simulink model "UniTire_0427_2021b_PID"  (R2021b)
settings: Solver=FixedStepAuto  StartTime=0.0  StopTime=15  FixedStep=0.001  RelTol=1e-3
model workspace (MAT data in the model file):
  v_obj = Simulink.Parameter
  v_obj.DataType = 'auto'
  v_obj.Complexity = 'real'
  v_obj.Dimensions = [0 0]
libraries: Solver_SF x1, slpidlib x1
settings Model: Creator=11580  LastModifiedBy=user
settings SolverCC: ZeroCrossAlgorithm=Adaptive
settings DebuggingCC: IgnoredZcDiagnostic=none  UnconnectedInputMsg=none  UnconnectedOutputMsg=none  UnconnectedLineMsg=none
settings ModelReferenceCC: EnableRefExpFcnMdlSchedulingChecks=off
settings RTWCC: DLArmComputeVersion=20.02.1

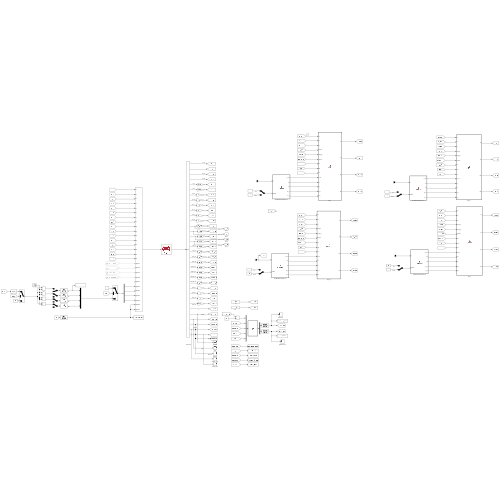
[thumbnail: Simulink's stored preview of the top-level diagram]
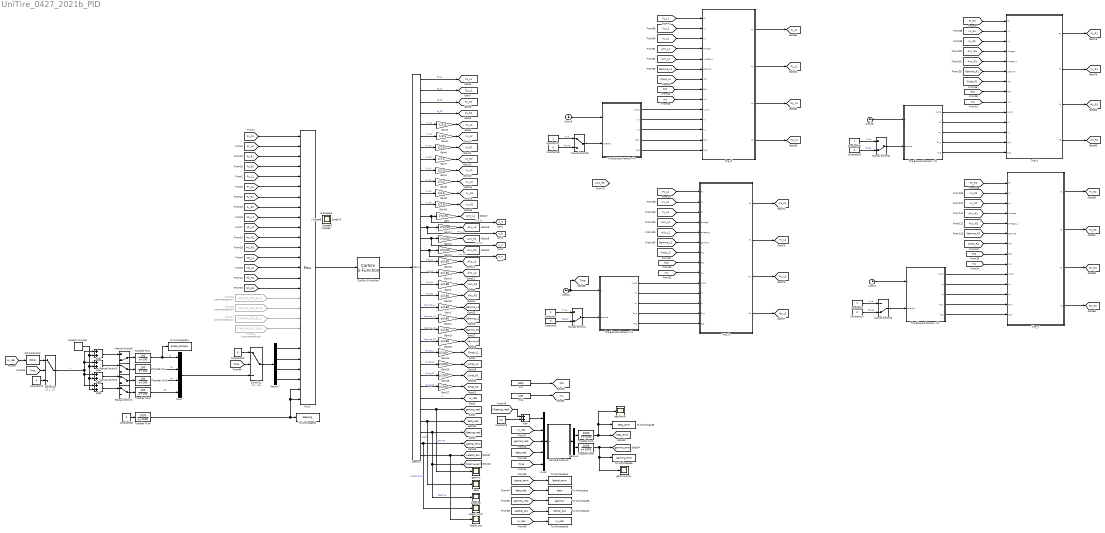
== system UniTire_0427_2021b_PID ==
  Add{,1..4} (5 alike) : Sum
  CarSim S-Function : Solver_SF/CarSim S-Function  Priority=1  SIMFILE=simfile.sim  Run_RTs=off  vs_state_ind=Run  StopMode_ind=Vehicle Model
  Clock{1..2,8..9} (4 alike) : Clock
  Constant{1..2,15,17} (4 alike) : Constant
  Constant{3,10,16,18,20..21,25} (7 alike) : Constant  Value=0
  Constant9 : Constant  Value=0.2
  Demux : Demux  Outputs=34
      settings: DisplayOption=none
  Demux1 : Demux  Outputs=2
  Demux7 : Demux
  From12 : From  Commented=on  GotoTag=IMP_MY_OUT_D2_R
  From17 : From  Commented=on  GotoTag=IMP_MY_OUT_D2_L
  From20 : From  Commented=on  GotoTag=IMP_MY_OUT_D1_R
  From21 : From  Commented=on  GotoTag=IMP_MY_OUT_D1_L
  Fzn : Constant  Value=4820
  Gain{,11..13} (4 alike) : Gain  Gain=2*pi/60
  Gain{1..2,14..19} (8 alike) : Gain  Gain=pi/180
  Gain{3..10} (8 alike) : Gain  Gain=1/3.6
  Gain{24..27} (4 alike) : Gain  Gain=1/1000
  MATLAB Function : MATLAB Function  TreatAsAtomicUnit=on
  Manual Switch{1,5..6,8} (4 alike) : ManualSwitch  CurrentSetting=0
  Manual Switch{2..4,9} (4 alike) : ManualSwitch
  Mux2 : Mux  Inputs=27
      settings: DisplayOption=signals
  Mux5 : Mux  Inputs=5
  Mux7 : Mux
  PID Controller : slpidlib/PID Controller  Controller=PID  Form=Parallel  TimeDomain=Continuous-time  UseExternalTs=off  SampleTime=-1  IntegratorMethod=Forward Euler  FilterMethod=Forward Euler  ControllerParametersSource=internal  P=4  I=0  D=1  UseFilter=on  N=100  TunerSelectOption=Transfer Function Based (PID Tuner App)  InitialConditionSource=internal  InitialConditionForIntegrator=0  InitialConditionForFilter=0  DifferentiatorICPrevScaledInput=0  ExternalReset=none  TrackingMode=off  Kt=1  LimitOutput=off  SatLimitsSource=internal  UpperSaturationLimit=inf  LowerSaturationLimit=-inf  LinearizeAsGain=on  AntiWindupMode=none  Kb=1  POutMin=[]  POutMax=[]  IOutMin=[]  IOutMax=[]  DOutMin=[]  DOutMax=[]  NOutMin=[]  NOutMax=[]  SumOutMin=[]  SumOutMax=[]  SaturationOutMin=[]  SaturationOutMax=[]  PParamMin=[]  PParamMax=[]  IParamMin=[]  IParamMax=[]  DParamMin=[]  DParamMax=[]  NParamMin=[]  NParamMax=[]  KbParamMin=[]  KbParamMax=[]  KtParamMin=[]  KtParamMax=[]  KbOutMin=[]  KbOutMax=[]  KtOutMin=[]  KtOutMax=[]  IntegratorOutMin=[]  IntegratorOutMax=[]  FilterOutMin=[]  FilterOutMax=[]  SumI1OutMin=[]  SumI1OutMax=[]  SumI2OutMin=[]  SumI2OutMax=[]  SumI3OutMin=[]  SumI3OutMax=[]  SumI4OutMin=[]  SumI4OutMax=[]  SumDOutMin=[]  SumDOutMax=[]  DifferentiatorOutMin=[]  DifferentiatorOutMax=[]  FilterDiffOutCoefMin=[]  FilterDiffOutCoefMax=[]  ReciprocalOutMin=[]  ReciprocalOutMax=[]  SumDenOutMin=[]  SumDenOutMax=[]  SumNumOutMin=[]  SumNumOutMax=[]  DivideOutMin=[]  DivideOutMax=[]  UdiffTsProdOutMin=[]  UdiffTsProdOutMax=[]  NTsProdOutMin=[]  NTsProdOutMax=[]  UintegralTsProdOutMin=[]  UintegralTsProdOutMax=[]  UngainTsProdOutMin=[]  UngainTsProdOutMax=[]  IntegratorContinuousStateAttributes=''  IntegratorStateMustResolveToSignalObject=off  IntegratorRTWStateStorageClass=Auto  FilterContinuousStateAttributes=''  FilterStateMustResolveToSignalObject=off  FilterRTWStateStorageClass=Auto  ParallelPVariant=InternalParameters  IdealPVariant=Disabled  IVariant=InternalParameters  DVariant=InternalParameters  IntegratorVariant=Continuous  SatVariant=Disabled  AWVariant=Passthrough  PCopyVariant=Disabled  TRVariant=Disabled  FdbkBlocksVariant=Forward  IdealPFdbkVariant=Disabled  SatFdbkVariant=Disabled  DerivativeFilterVariant=ContFilter  NVariant=InternalParameters  NCopyVariant=Disabled  FilterICVariant=InternalICsFilter  IntegratorICVariant=InternalICs  ExternalResetVariant=Disabled  TRSumVariant=Passthrough  SumFdbkVariant=Disabled  SumVariant=Sum_PID  TsampFilterVariant=InternalTs  TsampNgainVariant=Passthrough  TsampIntegralVariant=Passthrough  ExternalSaturationOutDataTypeStr=Inherit: Same as second input
  Random Number : RandomNumber  Variance=150  SampleTime=0.01
  Switch10 : Switch  Criteria=u2 > Threshold  Threshold=1.5
  Switch11 : Switch  Criteria=u2 > Threshold  Threshold=15
  Tire Blowout Params. rl1 : MATLAB Function  TreatAsAtomicUnit=on
  Tire Blowout Params. rl2 : MATLAB Function  TreatAsAtomicUnit=on
  Tire Blowout Params. rl3 : MATLAB Function  TreatAsAtomicUnit=on
  Tire Blowout Params. rl4 : MATLAB Function  TreatAsAtomicUnit=on
  Tire_fl : MATLAB Function  TreatAsAtomicUnit=on
  Tire_fr : MATLAB Function  TreatAsAtomicUnit=on
  Tire_rl1 : MATLAB Function  TreatAsAtomicUnit=on
  Tire_rr : MATLAB Function  TreatAsAtomicUnit=on
  To Workspace : ToWorkspace  VariableName=beta  SaveFormat=Timeseries  SampleTime=-1
  To Workspace1 : ToWorkspace  VariableName=lateral_error  SaveFormat=Timeseries  SampleTime=-1
  To Workspace11 : ToWorkspace  VariableName=Brake_torque1  SaveFormat=Timeseries  SampleTime=-1
  To Workspace2 : ToWorkspace  VariableName=Steering  SaveFormat=Timeseries  SampleTime=-1
  To Workspace3 : ToWorkspace  VariableName=gamma  SaveFormat=Timeseries  SampleTime=-1
  To Workspace4 : ToWorkspace  VariableName=lateral_acc  SaveFormat=Timeseries  SampleTime=-1
  To Workspace5 : ToWorkspace  VariableName=vx_real  SaveFormat=Timeseries  SampleTime=-1
  To Workspace8 : ToWorkspace  VariableName=beta_error  SaveFormat=Timeseries  SampleTime=-1
  To Workspace9 : ToWorkspace  VariableName=gamma_error  SaveFormat=Timeseries  SampleTime=-1
  Transfer Fcn{,1..3} (4 alike) : TransferFcn  Numerator=[100]  Denominator=[1 100]
  Transfer Fcn4 : TransferFcn  Numerator=[1000]  Denominator=[1 1000]
  Transfer Fcn5 : TransferFcn  Numerator=[1000]  Denominator=[1 1000]
  Transfer Fcn6 : TransferFcn  Numerator=[1000]  Denominator=[1 1000]
  beta : Scope
  beta error : Scope
  gamma : Scope
  gamma error : Scope
  lateral_acc : Scope
  lateral_error : Scope
  mu1 : Constant  Value=0.85
  steering : Scope
  Scope{,1..9,11..12,14,16,19..23,25..26} (21 alike) : Scope
  tag scope: AVy_L1=global, AVy_L2=global, AVy_R1=global, AVy_R2=global, AVz_L1=global, AVz_L2=global, AVz_R1=global, AVz_R2=global, Cmpt_L1=global, Cmpt_L2=global, Cmpt_R1=global, Cmpt_R2=global, Fx_L1=global, Fx_L2=global, Fx_R1=global, Fx_R2=global, Fy_L1=global, Fy_L2=global, Fy_R1=global, Fy_R2=global, Fz0=global, Fz_L1=global, Fz_L2=global, Fz_R1=global, Fz_R2=global, Gamma_L1=global, Gamma_L2=global, Gamma_R1=global, Gamma_R2=global, Lateral_acc=global, Lateral_error=global, My_L1=global, My_L2=global, My_R1=global, My_R2=global, Mz_L1=global, Mz_L2=global, Mz_R1=global, Mz_R2=global, Steering_real=global, Time=global, Vx_L1=global, Vx_L2=global, Vx_R1=global, Vx_R2=global, Vy_L1=global, Vy_L2=global, Vy_R1=global, Vy_R2=global, beta_error=global, beta_real=global, gamma_error=global, gamma_real=global, mu=global, n_fl=global, n_fr=global, n_rl=global, n_rr=global, vx_real=global
  wires:
  Demux/5 -> Gain3/1  "Vx_L1"
  Demux/13 -> [n_fl], Gain/1  "AVy_L1"
  Demux/17 -> Gain15/1  "AVz_L1"
  Demux/21 -> Gain1/1  "Gamma_L1"
  Demux/25 -> Gain24/1  "Cmpt_L1"
  Gain3/1 -> [Vx_L1]
  Demux/1 -> [Fz_L1]  "Fz_L1"
  Demux/2 -> [Fz_L2]  "Fz_L2"
  Demux/3 -> [Fz_R1]  "Fz_R1"
  Demux/4 -> [Fz_R2]  "Fz_R2"
  Demux/6 -> Gain5/1  "Vx_L2"
  Gain5/1 -> [Vx_L2]
  Demux/7 -> Gain6/1  "Vx_R1"
  Gain6/1 -> [Vx_R1]
  Demux/8 -> Gain7/1  "Vx_R2"
  Gain7/1 -> [Vx_R2]
  Gain4/1 -> [Vy_L1]
  Demux/9 -> Gain4/1  "Vy_L1"
  Gain8/1 -> [Vy_L2]
  Demux/10 -> Gain8/1  "Vy_L2"
  Gain9/1 -> [Vy_R1]
  Demux/11 -> Gain9/1  "Vy_R1"
  Gain10/1 -> [Vy_R2]
  Demux/12 -> Gain10/1  "Vy_R2"
  Gain/1 -> [AVy_L1]
  Gain11/1 -> [AVy_L2]
  Demux/14 -> [n_fr], Gain11/1  "AVy_L2"
  Gain12/1 -> [AVy_R1]
  Demux/15 -> [n_rl], Gain12/1  "AVy_R1"
  Gain13/1 -> [AVy_R2]
  Demux/16 -> [n_rr], Gain13/1  "AVy_R2"
  Demux/18 -> Gain14/1  "AVz_L2"
  Demux/19 -> Gain2/1  "AVz_R1"
  Demux/20 -> Gain16/1  "AVz_R2"
  Gain16/1 -> [AVz_R2]
  Gain1/1 -> [Gamma_L1]
  Gain17/1 -> [Gamma_L2]
  Demux/22 -> Gain17/1  "Gamma_L2"
  Gain18/1 -> [Gamma_R1]
  Demux/23 -> Gain18/1  "Gamma_R1"
  Gain19/1 -> [Gamma_R2]
  Demux/24 -> Gain19/1  "Gamma_R2"
  Gain2/1 -> [AVz_R1]
  Gain14/1 -> [AVz_L2]
  Gain15/1 -> [AVz_L1]
  Demux/26 -> Gain25/1  "Cmpt_21"
  Demux/27 -> Gain26/1  "Cmpt_R1"
  Demux/28 -> Gain27/1  "Cmpt_R2"
  Demux/29 -> [vx_real]  "Vx"
  [mu] -> Tire_rl1/9(mu)
  [Fz0] -> Tire_fr/8(Fz0)
  [Gamma_R1] -> Tire_fr/6(gamma)
  Tire_fr/4(Mz) -> [Mz_R1]
  [Fz_L1] -> Tire_fl/1(Fz)
  mu1/1 -> [mu]
  Tire_rl1/3(My) -> [My_L2]
  [AVy_L2] -> Tire_rl1/4(Omega)
  [AVz_R2] -> Tire_rr/5(omega_z)
  [Fz0] -> Tire_rr/8(Fz0)
  Fzn/1 -> [Fz0]
  [Gamma_R2] -> Tire_rr/6(gamma)
  Tire_fr/1(Fx) -> [Fx_R1]
  [Vx_R1] -> Tire_fr/2(Vx)
  [AVy_R2] -> Tire_rr/4(Omega)
  Tire_rr/1(Fx) -> [Fx_R2]
  Tire_rl1/4(Mz) -> [Mz_L2]
  [mu] -> Tire_rr/9(mu)
  [Cmpt_R2] -> Tire_rr/7(rho)
  [Vx_L2] -> Tire_rl1/2(Vx)
  Tire_fl/4(Mz) -> [Mz_L1]
  [Vx_R2] -> Tire_rr/2(Vx)
  [AVz_L2] -> Tire_rl1/5(omega_z)
  [mu] -> Tire_fl/9(mu)
  [AVz_L1] -> Tire_fl/5(omega_z)
  [Gamma_L1] -> Tire_fl/6(gamma)
  [AVy_R1] -> Tire_fr/4(Omega)
  Tire_rr/3(My) -> [My_R2]
  [Fz_R1] -> Tire_fr/1(Fz)
  [Gamma_L2] -> Tire_rl1/6(gamma)
  Tire_rr/4(Mz) -> [Mz_R2]
  [Cmpt_L2] -> Tire_rl1/7(rho)
  Tire_fl/3(My) -> [My_L1]
  [Fz0] -> Tire_rl1/8(Fz0)
  Tire_rl1/1(Fx) -> [Fx_L2]
  Tire_fl/1(Fx) -> [Fx_L1]
  [mu] -> Tire_fr/9(mu)
  [Fz_L2] -> Tire_rl1/1(Fz)
  [Vy_L2] -> Tire_rl1/3(Vy)
  [Fz_R2] -> Tire_rr/1(Fz)
  Tire_fr/3(My) -> [My_R1]
  [Vy_R1] -> Tire_fr/3(Vy)
  [Vy_R2] -> Tire_rr/3(Vy)
  [AVz_R1] -> Tire_fr/5(omega_z)
  [Fz0] -> Tire_fl/8(Fz0)
  [Cmpt_L1] -> Tire_fl/7(rho)
  [Cmpt_R1] -> Tire_fr/7(rho)
  [AVy_L1] -> Tire_fl/4(Omega)
  [Vy_L1] -> Tire_fl/3(Vy)
  From21/1 -> Mux2/17
  [My_R1] -> Mux2/11
  From12/1 -> Mux2/20
  [Mz_R2] -> Mux2/16
  [My_L2] -> Mux2/10
  [Fx_L2] -> Mux2/2
  [Fx_R2] -> Mux2/4
  [Fy_L1] -> Mux2/5
  [Fy_R1] -> Mux2/7
  [Fy_R2] -> Mux2/8
  [My_L1] -> Mux2/9
  [My_R2] -> Mux2/12
  [Mz_L2] -> Mux2/14
  [Fx_R1] -> Mux2/3
  From20/1 -> Mux2/18
  [Mz_R1] -> Mux2/15
  [Mz_L1] -> Mux2/13
  From17/1 -> Mux2/19
  [Fy_L2] -> Mux2/6
  [Fx_L1] -> Mux2/1
  [Vx_L1] -> Tire_fl/2(Vx)
  Gain24/1 -> [Cmpt_L1]
  Gain25/1 -> [Cmpt_L2]
  Gain26/1 -> [Cmpt_R1]
  Gain27/1 -> [Cmpt_R2]
  Tire Blowout Params. rl2/5(R_e) -> Tire_rr/14(R_e)
  Tire Blowout Params. rl2/4(Rr_c) -> Tire_rr/13(Rr_c)
  Tire Blowout Params. rl2/3(Ky) -> Tire_rr/12(Ky)
  Tire Blowout Params. rl2/2(Kx) -> Tire_rr/11(Kx)
  Tire Blowout Params. rl2/1(K_rho) -> Tire_rr/10(K_rho)
  Constant1/1 -> Manual Switch5/1  "True"
  Clock1/1 -> Tire Blowout Params. rl2/1(t)
  Constant10/1 -> Manual Switch5/2  "fause"
  Manual Switch5/1 -> Tire Blowout Params. rl2/2(enable)
  Manual Switch8/1 -> Tire Blowout Params. rl3/2(enable)
  Constant16/1 -> Manual Switch8/2  "fause"
  Clock8/1 -> Tire Blowout Params. rl3/1(t)
  Constant15/1 -> Manual Switch8/1  "True"
  Tire Blowout Params. rl3/1(K_rho) -> Tire_fr/10(K_rho)
  Tire Blowout Params. rl3/2(Kx) -> Tire_fr/11(Kx)
  Tire Blowout Params. rl3/3(Ky) -> Tire_fr/12(Ky)
  Tire Blowout Params. rl3/4(Rr_c) -> Tire_fr/13(Rr_c)
  Tire Blowout Params. rl3/5(R_e) -> Tire_fr/14(R_e)
  Tire Blowout Params. rl4/5(R_e) -> Tire_fl/14(R_e)
  Tire Blowout Params. rl4/4(Rr_c) -> Tire_fl/13(Rr_c)
  Tire Blowout Params. rl4/3(Ky) -> Tire_fl/12(Ky)
  Tire Blowout Params. rl4/2(Kx) -> Tire_fl/11(Kx)
  Tire Blowout Params. rl4/1(K_rho) -> Tire_fl/10(K_rho)
  Constant17/1 -> Manual Switch9/1  "True"
  Clock9/1 -> Tire Blowout Params. rl4/1(t)
  Constant18/1 -> Manual Switch9/2  "fause"
  Manual Switch9/1 -> Tire Blowout Params. rl4/2(enable)
  Manual Switch1/1 -> Tire Blowout Params. rl1/2(enable)
  Constant3/1 -> Manual Switch1/2  "fause"
  Clock2/1 -> [Time], Tire Blowout Params. rl1/1(t)
  Constant2/1 -> Manual Switch1/1  "True"
  Tire Blowout Params. rl1/1(K_rho) -> Tire_rl1/10(K_rho)
  Tire Blowout Params. rl1/2(Kx) -> Tire_rl1/11(Kx)
  Tire Blowout Params. rl1/3(Ky) -> Tire_rl1/12(Ky)
  Tire Blowout Params. rl1/4(Rr_c) -> Tire_rl1/13(Rr_c)
  Tire Blowout Params. rl1/5(R_e) -> Tire_rl1/14(R_e)
  Demux/30 -> [gamma_real], gamma/1  "gamma"
  Mux5/1 -> MATLAB Function/1(u)
  Demux/32 -> [Steering_real], steering/1, [Steering_real]  "steering"
  Demux/31 -> [beta_real], beta/1  "beta"
  [vx_real] -> Mux5/2
  [gamma_real] -> Mux5/3
  [beta_real] -> Mux5/4
  MATLAB Function/1(y) -> Demux1/1
  Demux1/1 -> Transfer Fcn5/1
  Demux1/2 -> Transfer Fcn6/1
  Demux/33 -> [Lateral_error], lateral_error/1  "lateral error"
  [Time] -> Switch10/2
  Demux/34 -> lateral_acc/1, [Lateral_acc]
  [beta_real] -> To Workspace/1
  [gamma_real] -> To Workspace3/1
  [Lateral_error] -> To Workspace1/1
  [Lateral_acc] -> To Workspace4/1
  [vx_real] -> To Workspace5/1
  Transfer Fcn/1 -> Mux7/2  "LR"
  Transfer Fcn1/1 -> Mux7/1, To Workspace11/1  "LF"
  Transfer Fcn2/1 -> Mux7/3  "RF"
  Transfer Fcn3/1 -> Mux7/4  "RR"
  Manual Switch2/1 -> Transfer Fcn3/1
  Manual Switch3/1 -> Transfer Fcn/1
  Manual Switch4/1 -> Transfer Fcn2/1
  Manual Switch6/1 -> Transfer Fcn1/1
  Mux7/1 -> Switch11/3
  [Time] -> Mux5/5
  Add/1 -> Mux5/1
  [Steering_real] -> Add/1
  Constant9/1 -> Add/2
  Transfer Fcn4/1 -> To Workspace2/1, Mux2/27, Mux2/26
  Transfer Fcn5/1 -> beta error/1, To Workspace8/1, [beta_error]
  Transfer Fcn6/1 -> To Workspace9/1, gamma error/1, [gamma_error]
  Tire_rl1/2(Fy) -> [Fy_L2]
  Tire_rr/2(Fy) -> [Fy_R2]
  Tire_fr/2(Fy) -> [Fy_R1]
  Tire_fl/2(Fy) -> [Fy_L1]
  [vx_real] -> PID Controller/1
  Mux2/1 -> CarSim S-Function/1
  CarSim S-Function/1 -> Demux/1
  Switch10/1 -> Add4/1, Add3/1, Add1/1, Add2/1  "1"
  PID Controller/1 -> Switch10/1
  Constant21/1 -> Switch10/3
  Add1/1 -> Manual Switch6/1
  Random Number/1 -> Add4/2, Add3/2, Add2/2, Add1/2
  Add2/1 -> Manual Switch3/1
  Add3/1 -> Manual Switch4/1
  Add4/1 -> Manual Switch2/1
  Demux7/1 -> Mux2/22
  Demux7/2 -> Mux2/23
  Demux7/3 -> Mux2/24
  Demux7/4 -> Mux2/25
  [Time] -> Switch11/2
  Constant20/1 -> Switch11/1
  Switch11/1 -> Demux7/1
  Constant25/1 -> Transfer Fcn4/1

== matlab function UniTire_0427_2021b_PID/Tire Blowout Params. rl4 ==
  data: K_rho output; Kx output; Ky output; Rr_c output; R_e output; t input; enable input
function [K_rho, Kx, Ky, Rr_c, R_e] = TireBlowout(t, enable)
% 初始参数
K_rho0 = 268000;     % Radial stiffness (N/m)
Kx0 = 1586.04;       % Longitudinal stiffness (N/unit slip)
Ky0 = 63430.51;      % Lateral stiffness (N/rad)
Rr_c0 = 0.0038;      % Rolling resistance coefficient
R_e0 = 0.325;        % Effective rolling radius

% 如果 enable<=0.5，始终输出初始参数
K_rho    = K_rho0;
Kx       = Kx0;
Ky       = Ky0;
Rr_c     = Rr_c0;
R_e      = R_e0;

   if enable > 0.5
       % 爆胎开始时间与过渡时长
       t_start    = 1;   % 3 s 开始
       t_duration = 0.1;   % 持续 100 ms
   
       % 计算过渡比例 t_ratio
       if     t <  t_start
              t_ratio = 0;
          elseif  t <= t_start + t_duration
              t_ratio = (t - t_start) / t_duration;
          else
              t_ratio = 1;    % 过渡完成后一直保持
       end
   
       % Define blowout parameter factors
       K_rho_factor    = 1/15;   % Reduce radial stiffness to 1/15
       Kx_factor       = 0.28;   % Reduce longitudinal stiffness to 28%
       Ky_factor       = 0.25;   % Reduce lateral stiffness to 25%
       Rr_c_factor     = 30;     % Increase rolling resistance by 30x
       R_e_factor      = 0.7;    % Reduce effective radius to 70%
   
       % 按 t_ratio 做线性插值
       K_rho    = K_rho0 * (1 - t_ratio) + (K_rho0 * K_rho_factor) * t_ratio;
       Kx       = Kx0 * (1 - t_ratio) + (Kx0 * Kx_factor) * t_ratio;
       Ky       = Ky0 * (1 - t_ratio) + (Ky0 * Ky_factor) * t_ratio;
       Rr_c     = Rr_c0 * (1 - t_ratio) + (Rr_c0 * Rr_c_factor) * t_ratio;
       R_e      = R_e0 * (1 - t_ratio) + (R_e0 * R_e_factor) * t_ratio;
   end

end

== matlab function UniTire_0427_2021b_PID/Tire_fl ==
  data: Fz input; Vx input; Fx output; Vy input; Omega input; omega_z input; gamma input; rho input; Fz0 input; mu input; K_rho input; Kx input; Ky input; Rr_c input; R_e input; Fy output; My output; Mz output
function [Fx, Fy, My, Mz] = UniTire_fl(Fz, Vx, Vy, Omega, omega_z, gamma, rho, Fz0, mu, K_rho, Kx, Ky, Rr_c, R_e)
%% 解析轮胎参数       
a1      = 0.02;  % 接地印迹半长经验系数1
a2      = 0.001; % 接地印迹半长经验系数2
lambda  = 1.00;  % 各向异性修正系数 
eps_val = 1e-12;
    
%% 计算
% 1.垂向力Fz
% Fz = K_rho * rho;
Fzn = Fz / Fz0; % 归一化垂向力

% 接地印迹半长
a = a1 * sqrt(max(Fz, 0)) + a2 * max(Fz, 0);

% 2.滑移率和刚度计算
    if abs(Omega) < eps_val
        Omega_safe = eps_val * sign(Omega + eps_val);  % Defaults to positive when Omega is exactly 0
    else
        Omega_safe = Omega;
    end

Sx = (Omega_safe * R_e - Vx) / (Omega_safe * R_e);  % 纵向滑移率
Sy = -Vy / (Omega_safe * R_e);                      % 侧向滑移率

%Sy_cam = -(Ky_gamma * sin(gamma)) / max(Ky, eps_val);
%Sy = Sy0 + Sy_cam; 

% 纵向及侧向的摩擦系数
%Ux = (Fzn^2 * (mu*(-0.048735)/0.345728)) + (Fzn*(mu*0.048084/0.345728)) + mu;
Ux = mu;
Uy = mu;

% 无量纲的相对滑移率
phi_X = (Sx * Kx) / max(Fz * Ux, eps_val);
phi_Y = (Sy * Ky) / max(Fz * Uy, eps_val);
phi = sqrt(phi_X.^2 + phi_Y.^2);

% 5.计算总切力因子 F
c1 = 15.804511^2; c2 = 13.644270^2; c3 = 132.496949; c4 = 8.120481;
E1 = 1 ./ ( exp(-Fzn / c1) * c2 + 2 );
Em = 1 ./ ( 2 + c3^2 * exp(-Fzn/c4^2) );

F = 1 - exp( -phi - ( phi^3 * (E1^2 + 1/12) + E1 * phi^2 ) );

% 计算纵向力部分
F_x = F * (phi_X / phi);
Fx = Fz * F_x * Ux;

% 计算侧向力部分
F_y = F * (phi_Y / phi);
Fy = Fz * F_y * Uy;

% 6.回正力矩计算
% 计算Kxc和Kyc
Kxc = 100548.546 * Fzn + 52024.374 * (Fzn^2); % 胎体纵向刚度 (N/m)
Kyc = 100548.546 * Fzn + 52024.374 * (Fzn^2); % 胎体侧向刚度 (N/m)

    % 限制最小刚度值
    Kxc = max(Kxc, 1000); % 最小刚度1kN/m
    Kyc = max(Kyc, 1000);
    
% 计算Dx参数
Dx0 = (-0.013812)*(Fzn^2) + 0.007221*Fzn - 0.025351;
De  = (-0.008474)*(Fzn^2) + 0.022706*Fzn - 0.005839;
D1 = 1.168453 * exp(-Fzn / 1.008694);  % 曲率因子1
D2 = 0.018910 * exp(-Fzn / 0.663584);  % 曲率因子2

% 回正力臂计算
lambda_d = 1 / (1 + (Ky/Kx) * (phi_Y/phi_X)^2);
Dx = (Dx0 - De) .* exp(-D1.*phi* lambda_d - D2.*(phi^2)) + De;

    % 限制Dx范围
    Dx = min(max(Dx, -0.1), 0.1); % 回正力臂应在±0.1m范围内

% 基本回正力矩计算MZ_base
Xc = Fx ./ max(Kxc, eps_val); 
Yc = Fy ./ max(Kyc, eps_val);

% 侧倾附加回正力矩Mxy
DeltaM_zm = abs( (5126.828074+84.910963.*Fzn+3846.585795*Fzn.^2) ).*Fz0;
Km_gamma = abs(Fz/(49.544278+(-56.993576*Fzn)+40.300204*Fzn.^2));    % 侧倾回正刚度 (Nm/rad)
phi_m = (Km_gamma / DeltaM_zm) * sin(gamma);
% 计算基准曲线Mxy_bar
DeltaMxy_bar = 1 - exp(-phi_m - Em*phi_m^2 - (Em^2 + 1/12)*phi_m^3);

% 侧倾附加回正力矩
    % 修正因子
    F_clipped = min(F, 1.0);
    lambda1 = sqrt(1 - F_clipped^2); 
    gamma_factor = 1 + 0.1*(gamma^2);
DeltaMz_gamma = gamma_factor * lambda1 * DeltaMxy_bar * DeltaM_zm;

% 总回正力矩
Mz = Fy.*Xc - Fx.*Yc + Fy.*Dx + DeltaMz_gamma;  

% 8.滚动阻力矩My
%Rr_c = 0.015; %滚动阻力系数
Rr_v = 0.000029;
My = Fz * (Rr_c + Rr_v * (Vy/3.6)) * R_e;
end

== matlab function UniTire_0427_2021b_PID/Tire_fr ==
  data: Fz input; Vx input; Fx output; Vy input; Omega input; omega_z input; gamma input; rho input; Fz0 input; mu input; K_rho input; Kx input; Ky input; Rr_c input; R_e input; Fy output; My output; Mz output
function [Fx, Fy, My, Mz] = UniTire_fr(Fz, Vx, Vy, Omega, omega_z, gamma, rho, Fz0, mu, K_rho, Kx, Ky, Rr_c, R_e)
%% 解析轮胎参数       
a1      = 0.02;  % 接地印迹半长经验系数1
a2      = 0.001; % 接地印迹半长经验系数2
lambda  = 1.00;  % 各向异性修正系数 
eps_val = 1e-12;
    
%% 计算
% 1.垂向力Fz
% Fz = K_rho * rho;
Fzn = Fz / Fz0; % 归一化垂向力

% 接地印迹半长
a = a1 * sqrt(max(Fz, 0)) + a2 * max(Fz, 0);

% 2.滑移率和刚度计算
    if abs(Omega) < eps_val
        Omega_safe = eps_val * sign(Omega + eps_val);  % Defaults to positive when Omega is exactly 0
    else
        Omega_safe = Omega;
    end

Sx = (Omega_safe * R_e - Vx) / (Omega_safe * R_e);  % 纵向滑移率
Sy = -Vy / (Omega_safe * R_e);                      % 侧向滑移率

%Sy_cam = -(Ky_gamma * sin(gamma)) / max(Ky, eps_val);
%Sy = Sy0 + Sy_cam; 

% 纵向及侧向的摩擦系数
%Ux = (Fzn^2 * (mu*(-0.048735)/0.345728)) + (Fzn*(mu*0.048084/0.345728)) + mu;
Ux = mu;
Uy = mu;

% 无量纲的相对滑移率
phi_X = (Sx * Kx) / max(Fz * Ux, eps_val);
phi_Y = (Sy * Ky) / max(Fz * Uy, eps_val);
phi = sqrt(phi_X.^2 + phi_Y.^2);

% 5.计算总切力因子 F
c1 = 15.804511^2; c2 = 13.644270^2; c3 = 132.496949; c4 = 8.120481;
E1 = 1 ./ ( exp(-Fzn / c1) * c2 + 2 );
Em = 1 ./ ( 2 + c3^2 * exp(-Fzn/c4^2) );

F = 1 - exp( -phi - ( phi^3 * (E1^2 + 1/12) + E1 * phi^2 ) );

% 计算纵向力部分
F_x = F * (phi_X / phi);
Fx = Fz * F_x * Ux;

% 计算侧向力部分
F_y = F * (phi_Y / phi);
Fy = Fz * F_y * Uy;

% 6.回正力矩计算
% 计算Kxc和Kyc
Kxc = 100548.546 * Fzn + 52024.374 * (Fzn^2); % 胎体纵向刚度 (N/m)
Kyc = 100548.546 * Fzn + 52024.374 * (Fzn^2); % 胎体侧向刚度 (N/m)

    % 限制最小刚度值
    Kxc = max(Kxc, 1000); % 最小刚度1kN/m
    Kyc = max(Kyc, 1000);
    
% 计算Dx参数
Dx0 = (-0.013812)*(Fzn^2) + 0.007221*Fzn - 0.025351;
De  = (-0.008474)*(Fzn^2) + 0.022706*Fzn - 0.005839;
D1 = 1.168453 * exp(-Fzn / 1.008694);  % 曲率因子1
D2 = 0.018910 * exp(-Fzn / 0.663584);  % 曲率因子2

% 回正力臂计算
lambda_d = 1 / (1 + (Ky/Kx) * (phi_Y/phi_X)^2);
Dx = (Dx0 - De) .* exp(-D1.*phi* lambda_d - D2.*(phi^2)) + De;

    % 限制Dx范围
    Dx = min(max(Dx, -0.1), 0.1); % 回正力臂应在±0.1m范围内

% 基本回正力矩计算MZ_base
Xc = Fx ./ max(Kxc, eps_val); 
Yc = Fy ./ max(Kyc, eps_val);

% 侧倾附加回正力矩Mxy
DeltaM_zm = abs( (5126.828074+84.910963.*Fzn+3846.585795*Fzn.^2) ).*Fz0;
Km_gamma = abs(Fz/(49.544278+(-56.993576*Fzn)+40.300204*Fzn.^2));    % 侧倾回正刚度 (Nm/rad)
phi_m = (Km_gamma / DeltaM_zm) * sin(gamma);
% 计算基准曲线Mxy_bar
DeltaMxy_bar = 1 - exp(-phi_m - Em*phi_m^2 - (Em^2 + 1/12)*phi_m^3);

% 侧倾附加回正力矩
    % 修正因子
    F_clipped = min(F, 1.0);
    lambda1 = sqrt(1 - F_clipped^2); 
    gamma_factor = 1 + 0.1*(gamma^2);
DeltaMz_gamma = gamma_factor * lambda1 * DeltaMxy_bar * DeltaM_zm;

% 总回正力矩
Mz = Fy.*Xc - Fx.*Yc + Fy.*Dx + DeltaMz_gamma;  

% 8.滚动阻力矩My
%Rr_c = 0.015; %滚动阻力系数
Rr_v = 0.000029;
My = Fz * (Rr_c + Rr_v * (Vy/3.6)) * R_e;
end

== matlab function UniTire_0427_2021b_PID/Tire_rr ==
  data: Fz input; Vx input; Fx output; Vy input; Omega input; omega_z input; gamma input; rho input; Fz0 input; mu input; K_rho input; Kx input; Ky input; Rr_c input; R_e input; Fy output; My output; Mz output
function [Fx, Fy, My, Mz] = UniTire_rr(Fz, Vx, Vy, Omega, omega_z, gamma, rho, Fz0, mu, K_rho, Kx, Ky, Rr_c, R_e)
%% 解析轮胎参数       
a1      = 0.02;  % 接地印迹半长经验系数1
a2      = 0.001; % 接地印迹半长经验系数2
lambda  = 1.00;  % 各向异性修正系数 
eps_val = 1e-12;
    
%% 计算
% 1.垂向力Fz
% Fz = K_rho * rho;
Fzn = Fz / Fz0; % 归一化垂向力

% 接地印迹半长
a = a1 * sqrt(max(Fz, 0)) + a2 * max(Fz, 0);

% 2.滑移率和刚度计算
    if abs(Omega) < eps_val
        Omega_safe = eps_val * sign(Omega + eps_val);  % Defaults to positive when Omega is exactly 0
    else
        Omega_safe = Omega;
    end

Sx = (Omega_safe * R_e - Vx) / (Omega_safe * R_e);  % 纵向滑移率
Sy = -Vy / (Omega_safe * R_e);                      % 侧向滑移率

%Sy_cam = -(Ky_gamma * sin(gamma)) / max(Ky, eps_val);
%Sy = Sy0 + Sy_cam; 

% 纵向及侧向的摩擦系数
%Ux = (Fzn^2 * (mu*(-0.048735)/0.345728)) + (Fzn*(mu*0.048084/0.345728)) + mu;
Ux = mu;
Uy = mu;

% 无量纲的相对滑移率
phi_X = (Sx * Kx) / max(Fz * Ux, eps_val);
phi_Y = (Sy * Ky) / max(Fz * Uy, eps_val);
phi = sqrt(phi_X.^2 + phi_Y.^2);

% 5.计算总切力因子 F
c1 = 15.804511^2; c2 = 13.644270^2; c3 = 132.496949; c4 = 8.120481;
E1 = 1 ./ ( exp(-Fzn / c1) * c2 + 2 );
Em = 1 ./ ( 2 + c3^2 * exp(-Fzn/c4^2) );

F = 1 - exp( -phi - ( phi^3 * (E1^2 + 1/12) + E1 * phi^2 ) );

% 计算纵向力部分
F_x = F * (phi_X / phi);
Fx = Fz * F_x * Ux;

% 计算侧向力部分
F_y = F * (phi_Y / phi);
Fy = Fz * F_y * Uy;

% 6.回正力矩计算
% 计算Kxc和Kyc
Kxc = 100548.546 * Fzn + 52024.374 * (Fzn^2); % 胎体纵向刚度 (N/m)
Kyc = 100548.546 * Fzn + 52024.374 * (Fzn^2); % 胎体侧向刚度 (N/m)

    % 限制最小刚度值
    Kxc = max(Kxc, 1000); % 最小刚度1kN/m
    Kyc = max(Kyc, 1000);
    
% 计算Dx参数
Dx0 = (-0.013812)*(Fzn^2) + 0.007221*Fzn - 0.025351;
De  = (-0.008474)*(Fzn^2) + 0.022706*Fzn - 0.005839;
D1 = 1.168453 * exp(-Fzn / 1.008694);  % 曲率因子1
D2 = 0.018910 * exp(-Fzn / 0.663584);  % 曲率因子2

% 回正力臂计算
lambda_d = 1 / (1 + (Ky/Kx) * (phi_Y/phi_X)^2);
Dx = (Dx0 - De) .* exp(-D1.*phi* lambda_d - D2.*(phi^2)) + De;

    % 限制Dx范围
    Dx = min(max(Dx, -0.1), 0.1); % 回正力臂应在±0.1m范围内

% 基本回正力矩计算MZ_base
Xc = Fx ./ max(Kxc, eps_val); 
Yc = Fy ./ max(Kyc, eps_val);

% 侧倾附加回正力矩Mxy
DeltaM_zm = abs( (5126.828074+84.910963.*Fzn+3846.585795*Fzn.^2) ).*Fz0;
Km_gamma = abs(Fz/(49.544278+(-56.993576*Fzn)+40.300204*Fzn.^2));    % 侧倾回正刚度 (Nm/rad)
phi_m = (Km_gamma / DeltaM_zm) * sin(gamma);
% 计算基准曲线Mxy_bar
DeltaMxy_bar = 1 - exp(-phi_m - Em*phi_m^2 - (Em^2 + 1/12)*phi_m^3);

% 侧倾附加回正力矩
    % 修正因子
    F_clipped = min(F, 1.0);
    lambda1 = sqrt(1 - F_clipped^2); 
    gamma_factor = 1 + 0.1*(gamma^2);
DeltaMz_gamma = gamma_factor * lambda1 * DeltaMxy_bar * DeltaM_zm;

% 总回正力矩
Mz = Fy.*Xc - Fx.*Yc + Fy.*Dx + DeltaMz_gamma;  

% 8.滚动阻力矩My
%Rr_c = 0.015; %滚动阻力系数
Rr_v = 0.000029;
My = Fz * (Rr_c + Rr_v * (Vy/3.6)) * R_e;
end

== matlab function UniTire_0427_2021b_PID/MATLAB Function ==
  data: u input; y output
function y = fcn(u)
delta_f = u(1) * pi / 180; % 前轮转角（单位：弧度）u1
v_x = u(2)/3.6;            % 纵向速度（单位：m/s） u2
gamma = u(3);
beta  = u(4);
time = u(5);
if time >1
    delta_f = delta_f - (0.2+0.574)* pi / 180;  % 0.574 RF
end
% if time >1
%     delta_f = delta_f - (-1.06 + 0.2)* pi / 180;  % 0.574 LF
% end
% if time >1
%     delta_f = delta_f - (0.141 + 0.2)* pi / 180;  % 0.574 LR
% end
% if time >1
%     delta_f = delta_f - (-0.657 + 0.2)* pi / 180;  % 0.574 RR
% end

l_f = 1.250;    % 前轴到质心距离（单位：m）
l_r = 1.400;    % 后轴到质心距离（单位：m）
m = 1750;       % 车辆质量（单位：kg）
K_r = 63430.51 * 2;    % 后轮侧偏刚度（单位：N/rad）
K_f = 63430.51 * 2;    % 后轮侧偏刚度（单位：N/rad）

L = l_f + l_r;
K = m * (l_f * K_f - l_r * K_r) / (K_f * K_r * (l_f + l_r)^2);
denominator = L * (1 + K * v_x^2);

% beta_r 计算 
numerator_beta = l_r + (m * l_f * v_x^2) / (K_r * L);
beta_r = (numerator_beta / denominator) * delta_f ;

% gamma_r 计算 
numerator_gamma = v_x / L;
gamma_r = (numerator_gamma / (1 + K * v_x^2)) * delta_f;

beta_e = beta-beta_r * 180 / pi;
gamma_e = gamma-gamma_r * 180 / pi;

y = [beta_e, gamma_e];

== matlab function UniTire_0427_2021b_PID/Tire_rl1 ==
  data: Fz input; Vx input; Fx output; Vy input; Omega input; omega_z input; gamma input; rho input; Fz0 input; mu input; K_rho input; Kx input; Ky input; Rr_c input; R_e input; Fy output; My output; Mz output
function [Fx, Fy, My, Mz] = UniTire_rl(Fz, Vx, Vy, Omega, omega_z, gamma, rho, Fz0, mu, K_rho, Kx, Ky, Rr_c, R_e)
%% 解析轮胎参数       
a1      = 0.02;  % 接地印迹半长经验系数1
a2      = 0.001; % 接地印迹半长经验系数2
lambda  = 1.00;  % 各向异性修正系数 
eps_val = 1e-12;
    
%% 计算
% 1.垂向力Fz
% Fz = K_rho * rho;
Fzn = Fz / Fz0; % 归一化垂向力

% 接地印迹半长
a = a1 * sqrt(max(Fz, 0)) + a2 * max(Fz, 0);

% 2.滑移率和刚度计算
    if abs(Omega) < eps_val
        Omega_safe = eps_val * sign(Omega + eps_val);  % Defaults to positive when Omega is exactly 0
    else
        Omega_safe = Omega;
    end

Sx = (Omega_safe * R_e - Vx) / (Omega_safe * R_e);  % 纵向滑移率
Sy = -Vy / (Omega_safe * R_e);                      % 侧向滑移率

%Sy_cam = -(Ky_gamma * sin(gamma)) / max(Ky, eps_val);
%Sy = Sy0 + Sy_cam; 

% 纵向及侧向的摩擦系数
%Ux = (Fzn^2 * (mu*(-0.048735)/0.345728)) + (Fzn*(mu*0.048084/0.345728)) + mu;
Ux = mu;
Uy = mu;

% 无量纲的相对滑移率
phi_X = (Sx * Kx) / max(Fz * Ux, eps_val);
phi_Y = (Sy * Ky) / max(Fz * Uy, eps_val);
phi = sqrt(phi_X.^2 + phi_Y.^2);

% 5.计算总切力因子 F
c1 = 15.804511^2; c2 = 13.644270^2; c3 = 132.496949; c4 = 8.120481;
E1 = 1 ./ ( exp(-Fzn / c1) * c2 + 2 );
Em = 1 ./ ( 2 + c3^2 * exp(-Fzn/c4^2) );

F = 1 - exp( -phi - ( phi^3 * (E1^2 + 1/12) + E1 * phi^2 ) );

% 计算纵向力部分
F_x = F * (phi_X / phi);
Fx = Fz * F_x * Ux;

% 计算侧向力部分
F_y = F * (phi_Y / phi);
Fy = Fz * F_y * Uy;

% 6.回正力矩计算
% 计算Kxc和Kyc
Kxc = 100548.546 * Fzn + 52024.374 * (Fzn^2); % 胎体纵向刚度 (N/m)
Kyc = 100548.546 * Fzn + 52024.374 * (Fzn^2); % 胎体侧向刚度 (N/m)

    % 限制最小刚度值
    Kxc = max(Kxc, 1000); % 最小刚度1kN/m
    Kyc = max(Kyc, 1000);
    
% 计算Dx参数
Dx0 = (-0.013812)*(Fzn^2) + 0.007221*Fzn - 0.025351;
De  = (-0.008474)*(Fzn^2) + 0.022706*Fzn - 0.005839;
D1 = 1.168453 * exp(-Fzn / 1.008694);  % 曲率因子1
D2 = 0.018910 * exp(-Fzn / 0.663584);  % 曲率因子2

% 回正力臂计算
lambda_d = 1 / (1 + (Ky/Kx) * (phi_Y/phi_X)^2);
Dx = (Dx0 - De) .* exp(-D1.*phi* lambda_d - D2.*(phi^2)) + De;

    % 限制Dx范围
    Dx = min(max(Dx, -0.1), 0.1); % 回正力臂应在±0.1m范围内

% 基本回正力矩计算MZ_base
Xc = Fx ./ max(Kxc, eps_val); 
Yc = Fy ./ max(Kyc, eps_val);

% 侧倾附加回正力矩Mxy
DeltaM_zm = abs( (5126.828074+84.910963.*Fzn+3846.585795*Fzn.^2) ).*Fz0;
Km_gamma = abs(Fz/(49.544278+(-56.993576*Fzn)+40.300204*Fzn.^2));    % 侧倾回正刚度 (Nm/rad)
phi_m = (Km_gamma / DeltaM_zm) * sin(gamma);
% 计算基准曲线Mxy_bar
DeltaMxy_bar = 1 - exp(-phi_m - Em*phi_m^2 - (Em^2 + 1/12)*phi_m^3);

% 侧倾附加回正力矩
    % 修正因子
    F_clipped = min(F, 1.0);
    lambda1 = sqrt(1 - F_clipped^2); 
    gamma_factor = 1 + 0.1*(gamma^2);
DeltaMz_gamma = gamma_factor * lambda1 * DeltaMxy_bar * DeltaM_zm;

% 总回正力矩
Mz = Fy.*Xc - Fx.*Yc + Fy.*Dx + DeltaMz_gamma;  

% 8.滚动阻力矩My
%Rr_c = 0.015; %滚动阻力系数
Rr_v = 0.000029;
My = Fz * (Rr_c + Rr_v * (Vy/3.6)) * R_e;
end

== matlab function UniTire_0427_2021b_PID/Tire Blowout Params. rl2 ==
  data: K_rho output; Kx output; Ky output; Rr_c output; R_e output; t input; enable input
function [K_rho, Kx, Ky, Rr_c, R_e] = TireBlowout(t, enable)
% 初始参数
K_rho0 = 268000;     % Radial stiffness (N/m)
Kx0 = 1586.04;       % Longitudinal stiffness (N/unit slip)
Ky0 = 63430.51;      % Lateral stiffness (N/rad)
Rr_c0 = 0.0038;      % Rolling resistance coefficient
R_e0 = 0.325;        % Effective rolling radius

% 如果 enable<=0.5，始终输出初始参数
K_rho    = K_rho0;
Kx       = Kx0;
Ky       = Ky0;
Rr_c     = Rr_c0;
R_e      = R_e0;

   if enable > 0.5
       % 爆胎开始时间与过渡时长
       t_start    = 1;   % 3 s 开始
       t_duration = 0.1;   % 持续 100 ms
   
       % 计算过渡比例 t_ratio
       if     t <  t_start
              t_ratio = 0;
          elseif  t <= t_start + t_duration
              t_ratio = (t - t_start) / t_duration;
          else
              t_ratio = 1;    % 过渡完成后一直保持
       end
   
       % Define blowout parameter factors
       K_rho_factor    = 1/15;   % Reduce radial stiffness to 1/15
       Kx_factor       = 0.28;   % Reduce longitudinal stiffness to 28%
       Ky_factor       = 0.25;   % Reduce lateral stiffness to 25%
       Rr_c_factor     = 30;     % Increase rolling resistance by 30x
       R_e_factor      = 0.7;    % Reduce effective radius to 70%
   
       % 按 t_ratio 做线性插值
       K_rho    = K_rho0 * (1 - t_ratio) + (K_rho0 * K_rho_factor) * t_ratio;
       Kx       = Kx0 * (1 - t_ratio) + (Kx0 * Kx_factor) * t_ratio;
       Ky       = Ky0 * (1 - t_ratio) + (Ky0 * Ky_factor) * t_ratio;
       Rr_c     = Rr_c0 * (1 - t_ratio) + (Rr_c0 * Rr_c_factor) * t_ratio;
       R_e      = R_e0 * (1 - t_ratio) + (R_e0 * R_e_factor) * t_ratio;
   end

end

== matlab function UniTire_0427_2021b_PID/Tire Blowout Params. rl1 ==
  data: K_rho output; Kx output; Ky output; Rr_c output; R_e output; t input; enable input
function [K_rho, Kx, Ky, Rr_c, R_e] = TireBlowout(t, enable)
% 初始参数
K_rho0 = 268000;     % Radial stiffness (N/m)
Kx0 = 1586.04;       % Longitudinal stiffness (N/unit slip)
Ky0 = 63430.51;      % Lateral stiffness (N/rad)
Rr_c0 = 0.0038;      % Rolling resistance coefficient
R_e0 = 0.325;        % Effective rolling radius

% 如果 enable<=0.5，始终输出初始参数
K_rho    = K_rho0;
Kx       = Kx0;
Ky       = Ky0;
Rr_c     = Rr_c0;
R_e      = R_e0;

   if enable > 0.5
       % 爆胎开始时间与过渡时长
       t_start    = 1;   % 3 s 开始
       t_duration = 0.1;   % 持续 100 ms
   
       % 计算过渡比例 t_ratio
       if     t <  t_start
              t_ratio = 0;
          elseif  t <= t_start + t_duration
              t_ratio = (t - t_start) / t_duration;
          else
              t_ratio = 1;    % 过渡完成后一直保持
       end
   
       % Define blowout parameter factors
       K_rho_factor    = 1/15;   % Reduce radial stiffness to 1/15
       Kx_factor       = 0.28;   % Reduce longitudinal stiffness to 28%
       Ky_factor       = 0.25;   % Reduce lateral stiffness to 25%
       Rr_c_factor     = 30;     % Increase rolling resistance by 30x
       R_e_factor      = 0.7;    % Reduce effective radius to 70%
   
       % 按 t_ratio 做线性插值
       K_rho    = K_rho0 * (1 - t_ratio) + (K_rho0 * K_rho_factor) * t_ratio;
       Kx       = Kx0 * (1 - t_ratio) + (Kx0 * Kx_factor) * t_ratio;
       Ky       = Ky0 * (1 - t_ratio) + (Ky0 * Ky_factor) * t_ratio;
       Rr_c     = Rr_c0 * (1 - t_ratio) + (Rr_c0 * Rr_c_factor) * t_ratio;
       R_e      = R_e0 * (1 - t_ratio) + (R_e0 * R_e_factor) * t_ratio;
   end

end

== matlab function UniTire_0427_2021b_PID/Tire Blowout Params. rl3 ==
  data: K_rho output; Kx output; Ky output; Rr_c output; R_e output; t input; enable input
function [K_rho, Kx, Ky, Rr_c, R_e] = TireBlowout(t, enable)
% 初始参数
K_rho0 = 268000;     % Radial stiffness (N/m)
Kx0 = 1586.04;       % Longitudinal stiffness (N/unit slip)
Ky0 = 63430.51;      % Lateral stiffness (N/rad)
Rr_c0 = 0.0038;      % Rolling resistance coefficient
R_e0 = 0.325;        % Effective rolling radius

% 如果 enable<=0.5，始终输出初始参数
K_rho    = K_rho0;
Kx       = Kx0;
Ky       = Ky0;
Rr_c     = Rr_c0;
R_e      = R_e0;

   if enable > 0.5
       % 爆胎开始时间与过渡时长
       t_start    = 1;   % 3 s 开始
       t_duration = 0.1;   % 持续 100 ms
   
       % 计算过渡比例 t_ratio
       if     t <  t_start
              t_ratio = 0;
          elseif  t <= t_start + t_duration
              t_ratio = (t - t_start) / t_duration;
          else
              t_ratio = 1;    % 过渡完成后一直保持
       end
   
       % Define blowout parameter factors
       K_rho_factor    = 1/15;   % Reduce radial stiffness to 1/15
       Kx_factor       = 0.28;   % Reduce longitudinal stiffness to 28%
       Ky_factor       = 0.25;   % Reduce lateral stiffness to 25%
       Rr_c_factor     = 30;     % Increase rolling resistance by 30x
       R_e_factor      = 0.7;    % Reduce effective radius to 70%
   
       % 按 t_ratio 做线性插值
       K_rho    = K_rho0 * (1 - t_ratio) + (K_rho0 * K_rho_factor) * t_ratio;
       Kx       = Kx0 * (1 - t_ratio) + (Kx0 * Kx_factor) * t_ratio;
       Ky       = Ky0 * (1 - t_ratio) + (Ky0 * Ky_factor) * t_ratio;
       Rr_c     = Rr_c0 * (1 - t_ratio) + (Rr_c0 * Rr_c_factor) * t_ratio;
       R_e      = R_e0 * (1 - t_ratio) + (R_e0 * R_e_factor) * t_ratio;
   end

end
